simulink model "Traffic_Light"  (R2022b)
settings: Solver=VariableStepAuto  StartTime=0.0  StopTime=10  RelTol=1e-3
settings Model: Creator=yasso  LastModifiedBy=yasso

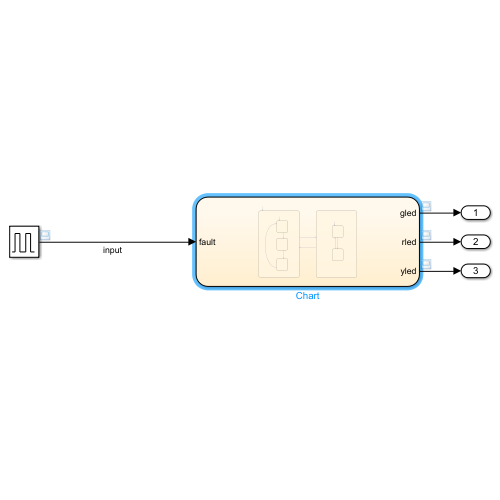
[thumbnail: Simulink's stored preview of the top-level diagram]
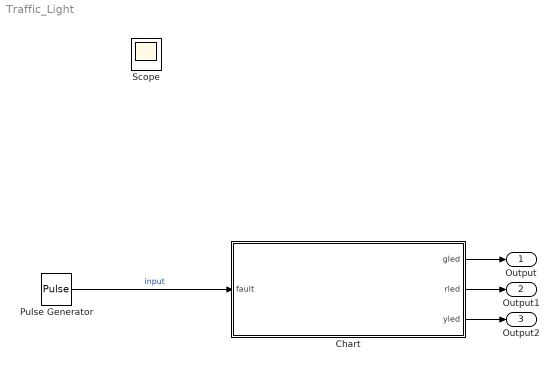
== system Traffic_Light ==
  Chart : Stateflow chart  TreatAsAtomicUnit=on
  Pulse Generator : DiscretePulseGenerator  PulseType=Time based  Period=10  PulseWidth=50
  Output : Outport
  Output1 : Outport  Port=2
  Output2 : Outport  Port=3
  Scope : Scope
  wires:
  Pulse Generator/1 -> Chart/1(fault)  "input"
  Chart/1(gled) -> Output/1
  Chart/2(rled) -> Output1/1
  Chart/3(yled) -> Output2/1

== stateflow chart Traffic_Light/Chart ==
  state normal
    state red
      en:
      rled=1
      gled=0
      yled=0
    state green
      en:
      rled=0
      gled=1
      yled=0
    state yellow
      en:
      rled=0
      gled=0
      yled=1
    (default) -> red
    yellow -> red : after(1,sec)
    red -> green : after(1,sec)
    green -> yellow : after(1,sec)
  state falier
    state on
      en:
      rled=1
    state off
      en:
      rled=0
    (default) -> on
    off -> on
    on -> off
  (default) -> normal
  normal -> falier : [fault ==1]
  falier -> normal : [fault==0]
  data: gled output; rled output; yled output; fault input
